simulink model "solucion_1_mat"  (R2020b)
settings: Solver=VariableStepAuto  StartTime=0.0  StopTime=10  RelTol=1e-3
model workspace (MAT data in the model file):
  Filter_span = 10
  Samples_per_symbol = 8
  Symbol_period = 2e-06
  alpha_fll = 0.392699081699
  gamma_fll = 0.01
  gamma_pll = 0.01
  phase_offset = 0
  ro_fll = 0.01
  ro_pll = 0.01
values from neighbouring files (symbols this model uses):
  doppler = [t', d']    [generate_doppler.m]
libraries: commutil2 x3, commsink2 x2, commchan3 x1, simulink x1, commdigbbndpm3 x1, commrandsrc3 x1
settings Model: Creator=Raul  LastModifiedBy=Raul
settings DataIOCC: ReturnWorkspaceOutputs=off

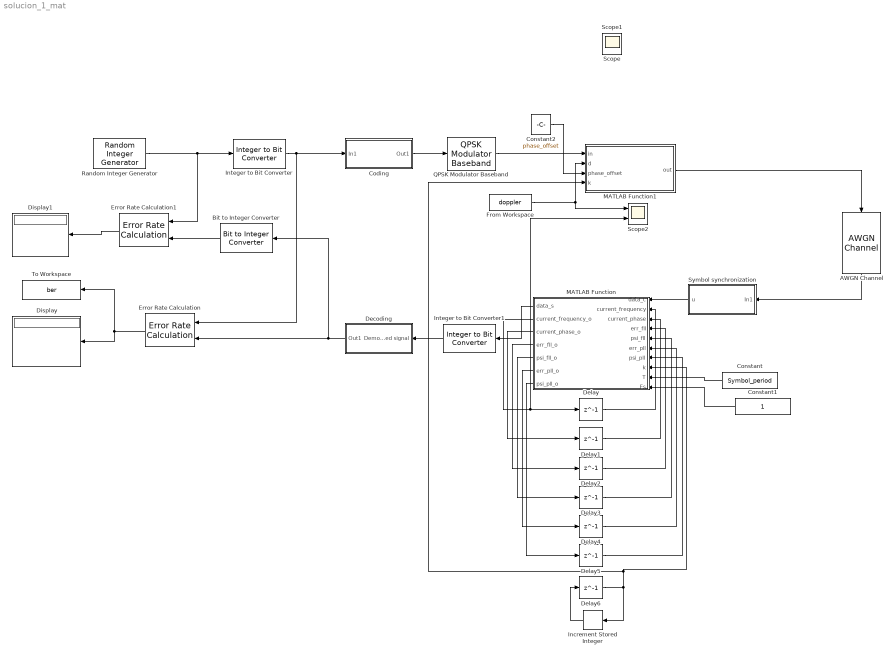
== system solucion_1_mat ==
  AWGN Channel : commchan3/AWGN Channel  InputProcessing=Columns as channels (frame based)  seed=57  noiseMode="Signal to noise ratio  (Eb/No)"  EbNodB=8  EsNodB=10  SNRdB=10  bitsPerSym=2  Ps=1  Tsym=Symbol_period  variance=1
  Bit to Integer Converter : commutil2/Bit to Integer Converter  nbits=2  bitOrder=MSB first  signedOutputValues=Unsigned  outDtype=Inherit via internal rule  outDtypeSigned=Inherit via internal rule
  Coding : Subsystem
  Constant : Constant  Value=Symbol_period
  Constant1 : Constant
  Constant2 : Constant  Value=phase_offset
  Decoding : Subsystem
  Delay : Delay  DelayLength=1  InitialCondition=doppler(1,2)
  Delay1 : Delay  DelayLength=1  InitialCondition=phase_offset
  Delay{2..6} (5 alike) : Delay  DelayLength=1  InitialCondition=0
  Display : Display
      settings: Format=short_e
  Display1 : Display
      settings: Format=short_e
  Error Rate Calculation : commsink2/Error Rate Calculation  N=0  st_delay=0  cp_mode=Entire frame  subframe=[]  PMode=Port  WsName=ErrorVec  RsMode2=off  stop=off  numErr=100  maxBits=1e6
  Error Rate Calculation1 : commsink2/Error Rate Calculation  N=0  st_delay=0  cp_mode=Entire frame  subframe=[]  PMode=Port  WsName=ErrorVec  RsMode2=off  stop=off  numErr=100  maxBits=1e6
  From Workspace : FromWorkspace  VariableName=doppler  SampleTime=-1  OutputAfterFinalValue=Holding final value
  Increment Stored Integer : simulink/Additional Math & Discrete/Additional Math: Increment - Decrement/Increment Stored Integer
  Integer to Bit Converter : commutil2/Integer to Bit Converter  nbits=2  signedInputValues=Unsigned  bitOrder=MSB first  outDtype=Inherit via internal rule
  Integer to Bit Converter1 : commutil2/Integer to Bit Converter  nbits=2  signedInputValues=Unsigned  bitOrder=LSB first  outDtype=uint8
  MATLAB Function : MATLAB Function  TreatAsAtomicUnit=on
  MATLAB Function1 : MATLAB Function  TreatAsAtomicUnit=on
  QPSK Modulator Baseband : commdigbbndpm3/QPSK Modulator Baseband  InType=Bit  Enc=Gray  Ph=pi/4  outDtype=double  outWordLen=16  outUDDataType=sfix(16)  outFracLenMode=Best precision  outFracLen=15  outDataTypeStr=double  outLastDataTypeStr=double
  Random Integer Generator : commrandsrc3/Random Integer Generator  SetSize=4  SeedSource=Parameter  Seed=456  SampleTime=Symbol_period  SamplesPerFrame=1  OutputDataType=uint8  SimulateUsing=Interpreted execution
  Scope2 : Scope  NumInputPorts=2
  Symbol synchronization : Subsystem
  To Workspace : ToWorkspace  VariableName=ber  SampleTime=-1
      settings: MaxDataPoints=1  Save2DSignal=2-D array (concatenate along first dimension)
  Scope : Scope
  Scope1 : Scope
  wires:
  Random Integer Generator/1 -> Error Rate Calculation1/1, Integer to Bit Converter/1
  Bit to Integer Converter/1 -> Error Rate Calculation1/2
  Integer to Bit Converter/1 -> Error Rate Calculation/1, Coding/1(In1)
  Error Rate Calculation/1 -> To Workspace/1, Display/1
  Error Rate Calculation1/1 -> Display1/1
  Coding/1(Out1) -> QPSK Modulator Baseband/1
  Decoding/1(Out1) -> Error Rate Calculation/2, Bit to Integer Converter/1
  Integer to Bit Converter1/1 -> Decoding/1(Demodulated signal)
  AWGN Channel/1 -> Symbol synchronization/1(In1)
  Symbol synchronization/1(u) -> MATLAB Function/1(data_c)
  MATLAB Function/1(data_s) -> Integer to Bit Converter1/1
  MATLAB Function/2(current_frequency_o) -> Delay/1, Scope2/2
  MATLAB Function/3(current_phase_o) -> Delay1/1
  MATLAB Function/4(err_fll_o) -> Delay2/1
  MATLAB Function/5(psi_fll_o) -> Delay3/1
  MATLAB Function/6(err_pll_o) -> Delay4/1
  MATLAB Function/7(psi_pll_o) -> Delay5/1
  Delay/1 -> MATLAB Function/2(current_frequency)
  Delay1/1 -> MATLAB Function/3(current_phase)
  Delay2/1 -> MATLAB Function/4(err_fll)
  Delay3/1 -> MATLAB Function/5(psi_fll)
  Delay4/1 -> MATLAB Function/6(err_pll)
  Delay5/1 -> MATLAB Function/7(psi_pll)
  Delay6/1 -> MATLAB Function1/4(k), MATLAB Function/8(k), Increment Stored Integer/1
  Increment Stored Integer/1 -> Delay6/1
  Constant/1 -> MATLAB Function/9(T)
  Constant1/1 -> MATLAB Function/10(Es)
  MATLAB Function1/1(out) -> AWGN Channel/1
  QPSK Modulator Baseband/1 -> MATLAB Function1/1(in)
  From Workspace/1 -> MATLAB Function1/2(d), Scope2/1
  Constant2/1 -> MATLAB Function1/3(phase_offset)

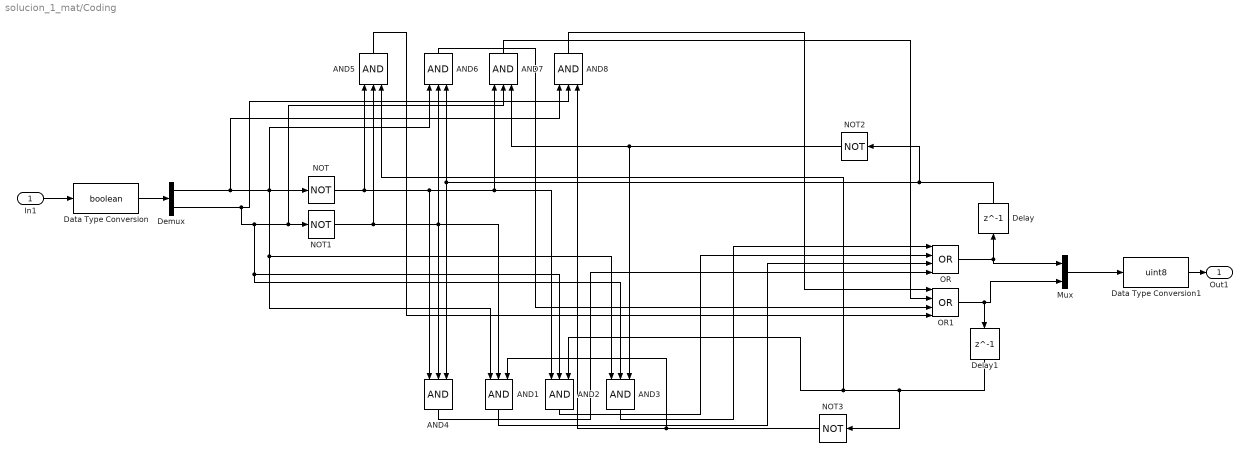
== system solucion_1_mat/Coding ==
  In1 : Inport
  AND{1..8} (8 alike) : Logic  Inputs=3  IconShape=distinctive  AllPortsSameDT=off  OutDataTypeStr=boolean
  Data Type Conversion : DataTypeConversion  OutDataTypeStr=boolean
  Data Type Conversion1 : DataTypeConversion  OutDataTypeStr=uint8
  Delay : Delay  DelayLength=1  InitialCondition=0
  Delay1 : Delay  DelayLength=1  InitialCondition=0
  Demux : Demux  Outputs=2
  Mux : Mux  Inputs=2
  NOT{,1..3} (4 alike) : Logic  Operator=NOT  IconShape=distinctive  AllPortsSameDT=off  OutDataTypeStr=boolean
  OR : Logic  Operator=OR  Inputs=4  IconShape=distinctive  AllPortsSameDT=off  OutDataTypeStr=boolean
  OR1 : Logic  Operator=OR  Inputs=4  IconShape=distinctive  AllPortsSameDT=off  OutDataTypeStr=boolean
  Out1 : Outport
  wires:
  Demux/1 -> AND8/1, AND6/1, AND3/1, AND1/1, NOT/1
  OR/1 -> Delay/1, Mux/1
  OR1/1 -> Mux/2, Delay1/1
  Delay/1 -> AND6/3, AND4/3, NOT2/1
  Demux/2 -> AND8/2, AND2/2, AND3/2, AND7/2, NOT1/1
  Delay1/1 -> NOT3/1, AND5/3, AND2/3
  NOT/1 -> AND7/1, AND2/1, AND4/1, AND5/1
  NOT1/1 -> AND6/2, AND1/2, AND4/2, AND5/2
  Mux/1 -> Data Type Conversion1/1
  NOT3/1 -> AND8/3, AND1/3
  NOT2/1 -> AND7/3, AND3/3
  AND3/1 -> OR/1
  AND2/1 -> OR/2
  AND1/1 -> OR/3
  AND4/1 -> OR/4
  AND8/1 -> OR1/1
  AND6/1 -> OR1/3
  AND7/1 -> OR1/2
  AND5/1 -> OR1/4
  Data Type Conversion/1 -> Demux/1
  In1/1 -> Data Type Conversion/1
  Data Type Conversion1/1 -> Out1/1

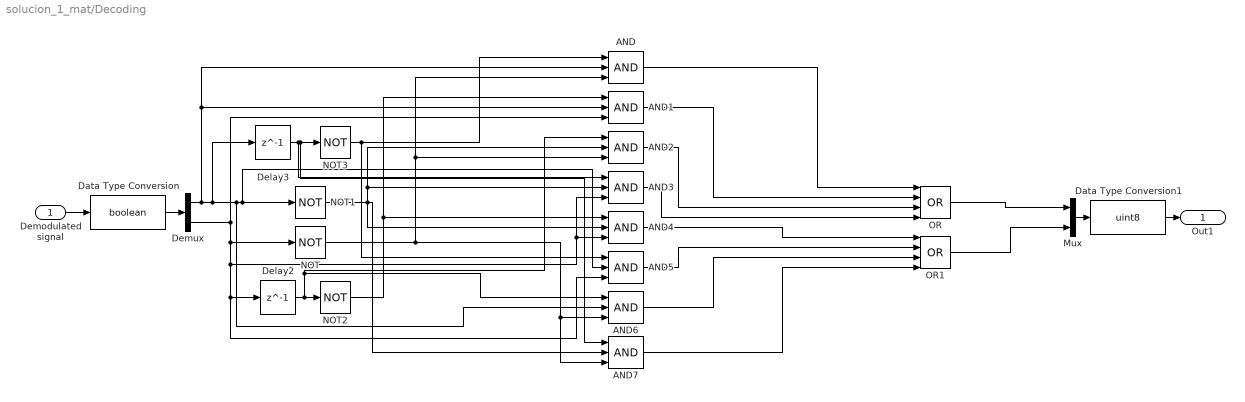
== system solucion_1_mat/Decoding ==
  Demodulated signal : Inport
  AND{,1..7} (8 alike) : Logic  Inputs=3  IconShape=distinctive  AllPortsSameDT=off  OutDataTypeStr=boolean
  Data Type Conversion : DataTypeConversion  OutDataTypeStr=boolean
  Data Type Conversion1 : DataTypeConversion  OutDataTypeStr=uint8
  Delay2 : Delay  DelayLength=1  InitialCondition=0
  Delay3 : Delay  DelayLength=1  InitialCondition=0
  Demux : Demux  Outputs=2
  Mux : Mux  Inputs=2
  NOT{,1..3} (4 alike) : Logic  Operator=NOT  IconShape=distinctive  AllPortsSameDT=off  OutDataTypeStr=boolean
  OR : Logic  Operator=OR  Inputs=4  IconShape=distinctive  AllPortsSameDT=off  OutDataTypeStr=boolean
  OR1 : Logic  Operator=OR  Inputs=4  IconShape=distinctive  AllPortsSameDT=off  OutDataTypeStr=boolean
  Out1 : Outport
  wires:
  OR/1 -> Mux/1
  Demux/2 -> AND4/3, AND3/3, AND5/3, Delay2/1, NOT/1, AND1/3
  Delay2/1 -> AND6/1, AND2/1, NOT2/1
  Demux/1 -> AND1/2, AND/2, Delay3/1, AND6/2, AND5/2, NOT1/1
  Delay3/1 -> AND3/1, AND7/1, NOT3/1
  AND7/1 -> OR1/4
  AND6/1 -> OR1/3
  AND5/1 -> OR1/2
  AND4/1 -> OR1/1
  AND/1 -> OR/1
  AND1/1 -> OR/2
  AND2/1 -> OR/3
  AND3/1 -> OR/4
  OR1/1 -> Mux/2
  NOT3/1 -> AND5/1, AND/1
  NOT/1 -> AND7/3, AND6/3, AND2/3, AND/3
  NOT2/1 -> AND4/1, AND1/1
  NOT1/1 -> AND7/2, AND3/2, AND2/2, AND4/2
  Demodulated signal/1 -> Data Type Conversion/1
  Data Type Conversion/1 -> Demux/1
  Mux/1 -> Data Type Conversion1/1
  Data Type Conversion1/1 -> Out1/1

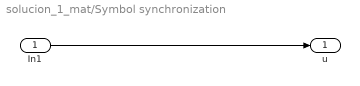
== system solucion_1_mat/Symbol synchronization ==
  In1 : Inport
  u : Outport  OutDataTypeStr=double
  wires:
  In1/1 -> u/1

== matlab function solucion_1_mat/MATLAB Function1 ==
  data: in input; d input; out output; phase_offset input; k input
function out = apply_doppler_and_phase(in, d,phase_offset,k)
    T = 2e-6;
    out = in * exp(1j*((2*pi*d.*k*T)+phase_offset));
end

== matlab function solucion_1_mat/MATLAB Function ==
  data: data_c input; data_s output; current_frequency input; current_phase input; err_fll input; psi_fll input; err_pll input; psi_pll input; current_frequency_o output; current_phase_o output; err_fll_o output; psi_fll_o output; err_pll_o output; psi_pll_o output; k input; T input; Es input
function [data_s,current_frequency_o, current_phase_o,err_fll_o,psi_fll_o,err_pll_o,psi_pll_o] = carrier_synchro(data_c,current_frequency, current_phase,err_fll,psi_fll,err_pll,psi_pll,k,T,Es)
    alpha_fll = pi/8;
    gamma_pll = 0.01;
    ro_pll = 0.01;
    gamma_fll = 0.01;
    ro_fll = 0.01;

    %FLL Detector
    q = data_c .* exp(-1j*(2*pi*k*T*current_frequency));
 
    est = sqrt(Es)*qpsk_modulator_custom_norm(qpsk_detector(q));
    
    
    %FLL error generator
    z_fll = angle(q*est');
    err_prev_fll = err_fll;
    if abs(z_fll) < alpha_fll
        err_fll = z_fll;
    end
    
    %FLL error filtering
    psi_prev_fll = psi_fll;
    psi_fll = psi_prev_fll + gamma_fll* (1+ro_fll) * err_fll - gamma_fll* err_prev_fll;
    
    
    % PLL Detector

    q = q .* exp(-1j*current_phase);
    
    data_s = qpsk_detector(q);
    
    est = sqrt(Es)*qpsk_modulator_custom_norm(data_s);
    
    % PLL detector
    err_prev_pll = err_pll;
    err_pll = imag(q*est');
    
    % PLL error filtering
    psi_prev_pll = psi_pll;
    psi_pll = psi_prev_pll + gamma_pll* (1+ro_pll) * err_pll - gamma_pll* err_prev_pll;
    

    %Updating the oscillator values
    current_frequency_o = current_frequency+psi_fll;
    current_phase_o = current_phase+psi_pll;
    err_fll_o = err_fll;
    err_pll_o = err_pll;
    psi_fll_o = psi_fll;
    psi_pll_o = psi_pll;

end
